simulink model "battery_convertidor_ac_dc_43"  (R2024b)
settings: Solver=FixedStepAuto  StartTime=0.0  StopTime=751  FixedStep=1e-5  RelTol=1e-3
InitFcn:
  | Tint = 1e-5;
  | Ts = 10*Tint;
values from neighbouring files (symbols this model uses):
  C1_filter = 20e-6    (= 2e-05)    [parametros_generales.m]
  I_control = 1    [parametros_generales.m]
  I_control_bat = 5    [parametros_generales.m]
  L_converter = 20e-3    (= 0.02)    [parametros_generales.m]
  Lbat_converter = 1e-5    (= 1e-05)    [parametros_generales.m]
  load_dc = 1000*1000/5    (= 200000)    [parametros_generales.m]
  P_control = 0.01    [parametros_generales.m]
  P_control_bat = 0.7    [parametros_generales.m]
  R = 0.5    [parametros_generales.m]
  R_filter = 0.5    [parametros_generales.m]
  rated_capacitance = 62.5/8    (= 7.8125)    [parametros_generales.m]
  rated_voltage = 144*8    (= 1152)    [parametros_generales.m]
  sample_time_control = 4e-4    (= 0.0004)    [parametros_generales.m]
  voltage_dc_source = 1000    [parametros_generales.m]
undefined symbols (not defined in the file or in its folder): Ion, Lithium
libraries: spsIGBTDiodeLib x24, spsCurrentMeasurementLib x23, spsSeriesRLCBranchLib x20, spsVoltageMeasurementLib x14, spsPower3phInstantaneousLib x8, spsThreePhaseVIMeasurementLib x8, simulink x7, dspstat3 x6, slpidlib x3, spsBatteryLib x2, spsVariableCapacitorLib x1, spsVariableResistorLib x1
(part 2 of 2)

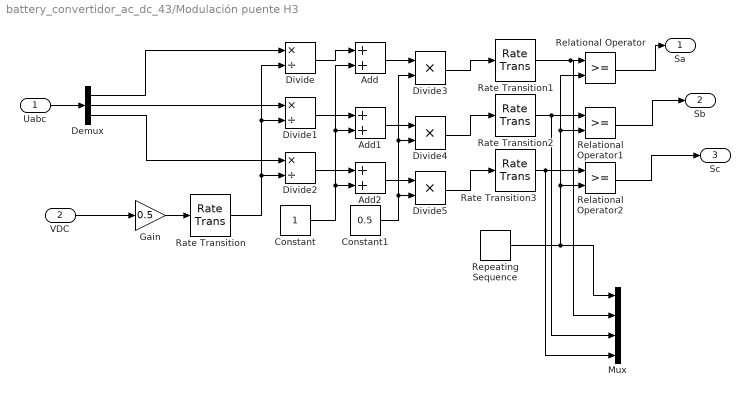
== system battery_convertidor_ac_dc_43/Modulación puente H3 ==
  Uabc : Inport
  VDC : Inport  Port=2
  Add : Sum
  Add1 : Sum
  Add2 : Sum
  Constant : Constant
  Constant1 : Constant  Value=0.5
  Demux : Demux  Outputs=3
  Divide : Product  Inputs=*/
  Divide1 : Product  Inputs=*/
  Divide2 : Product  Inputs=*/
  Divide3 : Product  Inputs=**
  Divide4 : Product  Inputs=**
  Divide5 : Product  Inputs=**
  Gain : Gain  Gain=0.5
  Mux : Mux
  Rate Transition : RateTransition  OutPortSampleTime=Ts
  Rate Transition1 : RateTransition  OutPortSampleTime=Tint
  Rate Transition2 : RateTransition  OutPortSampleTime=Tint
  Rate Transition3 : RateTransition  OutPortSampleTime=Tint
  Relational Operator : RelationalOperator  OutDataTypeStr=boolean  RndMeth=Simplest  InputSameDT=off
  Relational Operator1 : RelationalOperator  OutDataTypeStr=boolean  RndMeth=Simplest  InputSameDT=off
  Relational Operator2 : RelationalOperator  OutDataTypeStr=boolean  RndMeth=Simplest  InputSameDT=off
  Repeating Sequence : simulink/Sources/Repeating Sequence  rep_seq_t=[0 Ts/2 Ts]  rep_seq_y=[0 1 0]
  Sa : Outport
  Sb : Outport  Port=2
  Sc : Outport  Port=3
  wires:
  Demux/3 -> Divide2/1
  Demux/1 -> Divide/1
  Demux/2 -> Divide1/1
  Relational Operator/1 -> Sa/1
  Relational Operator1/1 -> Sb/1
  Relational Operator2/1 -> Sc/1
  Rate Transition/1 -> Divide1/2, Divide/2, Divide2/2
  Divide/1 -> Add/1
  Add/1 -> Divide3/1
  Divide3/1 -> Rate Transition1/1
  Add1/1 -> Divide4/1
  Add2/1 -> Divide5/1
  Divide1/1 -> Add1/1
  Divide4/1 -> Rate Transition2/1
  Divide2/1 -> Add2/1
  Divide5/1 -> Rate Transition3/1
  Constant/1 -> Add2/2, Add1/2, Add/2
  Constant1/1 -> Divide5/2, Divide4/2, Divide3/2
  Uabc/1 -> Demux/1
  Repeating Sequence/1 -> Mux/1, Relational Operator2/2, Relational Operator1/2, Relational Operator/2
  Rate Transition3/1 -> Mux/4, Relational Operator2/1
  Rate Transition2/1 -> Mux/3, Relational Operator1/1
  Rate Transition1/1 -> Mux/2, Relational Operator/1
  Gain/1 -> Rate Transition/1
  VDC/1 -> Gain/1

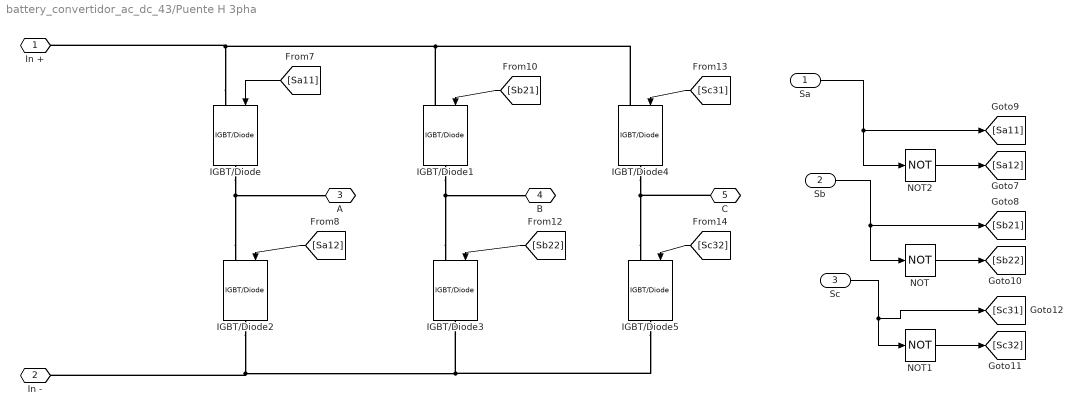
== system battery_convertidor_ac_dc_43/Puente H 3pha ==
  Sa : Inport
  Sb : Inport  Port=2
  Sc : Inport  Port=3
  IGBT/Diode{,1..5} (6 alike) : spsIGBTDiodeLib/IGBT//Diode  Ron=1e-3  Rs=1e5  Cs=inf  Measurements=off
  NOT : Logic  Operator=NOT  IconShape=distinctive  AllPortsSameDT=off  OutDataTypeStr=boolean
  NOT1 : Logic  Operator=NOT  IconShape=distinctive  AllPortsSameDT=off  OutDataTypeStr=boolean
  NOT2 : Logic  Operator=NOT  IconShape=distinctive  AllPortsSameDT=off  OutDataTypeStr=boolean
  In + : PMIOPort  Side=Left
  In - : PMIOPort  Port=2  Side=Left
  A : PMIOPort  Port=3  Side=Right
  B : PMIOPort  Port=4  Side=Right
  C : PMIOPort  Port=5  Side=Right
  wires:
  [Sa11] -> IGBT/Diode/1
  [Sc31] -> IGBT/Diode4/1
  [Sc32] -> IGBT/Diode5/1
  NOT2/1 -> [Sa12]
  NOT/1 -> [Sb22]
  [Sb21] -> IGBT/Diode1/1
  [Sa12] -> IGBT/Diode2/1
  [Sb22] -> IGBT/Diode3/1
  NOT1/1 -> [Sc32]
  Sa/1 -> [Sa11], NOT2/1
  Sb/1 -> [Sb21], NOT/1
  Sc/1 -> [Sc31], NOT1/1
  connections:
  IGBT/Diode2/LConn1 -- A/RConn1 -- IGBT/Diode/RConn1
  IGBT/Diode5/LConn1 -- C/RConn1 -- IGBT/Diode4/RConn1
  In -/RConn1 -- IGBT/Diode2/RConn1 -- IGBT/Diode5/RConn1 -- IGBT/Diode3/RConn1
  IGBT/Diode/LConn1 -- In +/RConn1 -- IGBT/Diode4/LConn1 -- IGBT/Diode1/LConn1
  IGBT/Diode3/LConn1 -- B/RConn1 -- IGBT/Diode1/RConn1

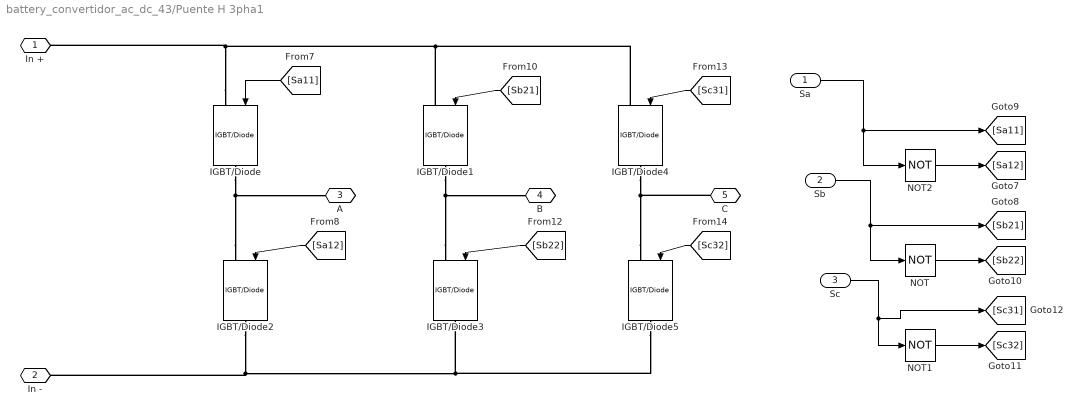
== system battery_convertidor_ac_dc_43/Puente H 3pha1 ==
  Sa : Inport
  Sb : Inport  Port=2
  Sc : Inport  Port=3
  IGBT/Diode{,1..5} (6 alike) : spsIGBTDiodeLib/IGBT//Diode  Ron=1e-3  Rs=1e5  Cs=inf  Measurements=off
  NOT : Logic  Operator=NOT  IconShape=distinctive  AllPortsSameDT=off  OutDataTypeStr=boolean
  NOT1 : Logic  Operator=NOT  IconShape=distinctive  AllPortsSameDT=off  OutDataTypeStr=boolean
  NOT2 : Logic  Operator=NOT  IconShape=distinctive  AllPortsSameDT=off  OutDataTypeStr=boolean
  In + : PMIOPort  Side=Left
  In - : PMIOPort  Port=2  Side=Left
  A : PMIOPort  Port=3  Side=Right
  B : PMIOPort  Port=4  Side=Right
  C : PMIOPort  Port=5  Side=Right
  wires:
  [Sa11] -> IGBT/Diode/1
  [Sc31] -> IGBT/Diode4/1
  [Sc32] -> IGBT/Diode5/1
  NOT2/1 -> [Sa12]
  NOT/1 -> [Sb22]
  [Sb21] -> IGBT/Diode1/1
  [Sa12] -> IGBT/Diode2/1
  [Sb22] -> IGBT/Diode3/1
  NOT1/1 -> [Sc32]
  Sa/1 -> [Sa11], NOT2/1
  Sb/1 -> [Sb21], NOT/1
  Sc/1 -> [Sc31], NOT1/1
  connections:
  IGBT/Diode2/LConn1 -- A/RConn1 -- IGBT/Diode/RConn1
  IGBT/Diode5/LConn1 -- C/RConn1 -- IGBT/Diode4/RConn1
  In -/RConn1 -- IGBT/Diode2/RConn1 -- IGBT/Diode5/RConn1 -- IGBT/Diode3/RConn1
  IGBT/Diode/LConn1 -- In +/RConn1 -- IGBT/Diode4/LConn1 -- IGBT/Diode1/LConn1
  IGBT/Diode3/LConn1 -- B/RConn1 -- IGBT/Diode1/RConn1

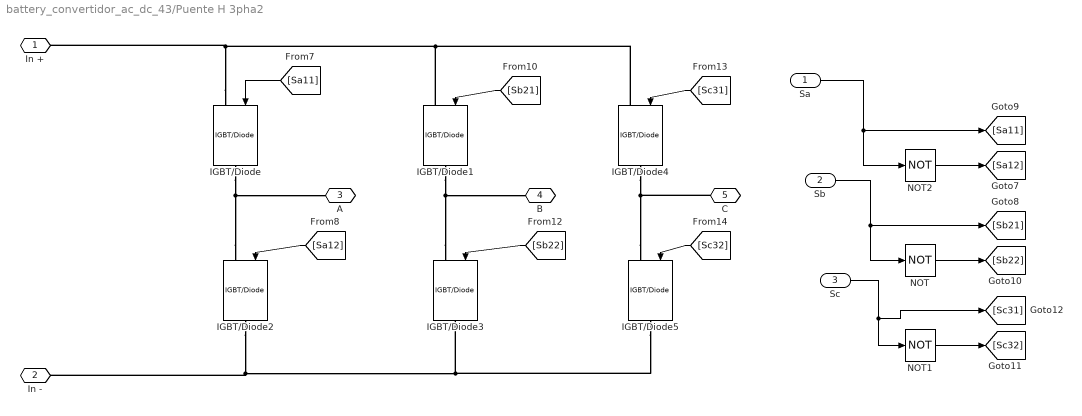
== system battery_convertidor_ac_dc_43/Puente H 3pha2 ==
  Sa : Inport
  Sb : Inport  Port=2
  Sc : Inport  Port=3
  IGBT/Diode{,1..5} (6 alike) : spsIGBTDiodeLib/IGBT//Diode  Ron=1e-3  Rs=1e5  Cs=inf  Measurements=off
  NOT : Logic  Operator=NOT  IconShape=distinctive  AllPortsSameDT=off  OutDataTypeStr=boolean
  NOT1 : Logic  Operator=NOT  IconShape=distinctive  AllPortsSameDT=off  OutDataTypeStr=boolean
  NOT2 : Logic  Operator=NOT  IconShape=distinctive  AllPortsSameDT=off  OutDataTypeStr=boolean
  In + : PMIOPort  Side=Left
  In - : PMIOPort  Port=2  Side=Left
  A : PMIOPort  Port=3  Side=Right
  B : PMIOPort  Port=4  Side=Right
  C : PMIOPort  Port=5  Side=Right
  wires:
  [Sa11] -> IGBT/Diode/1
  [Sc31] -> IGBT/Diode4/1
  [Sc32] -> IGBT/Diode5/1
  NOT2/1 -> [Sa12]
  NOT/1 -> [Sb22]
  [Sb21] -> IGBT/Diode1/1
  [Sa12] -> IGBT/Diode2/1
  [Sb22] -> IGBT/Diode3/1
  NOT1/1 -> [Sc32]
  Sa/1 -> [Sa11], NOT2/1
  Sb/1 -> [Sb21], NOT/1
  Sc/1 -> [Sc31], NOT1/1
  connections:
  IGBT/Diode2/LConn1 -- A/RConn1 -- IGBT/Diode/RConn1
  IGBT/Diode5/LConn1 -- C/RConn1 -- IGBT/Diode4/RConn1
  In -/RConn1 -- IGBT/Diode2/RConn1 -- IGBT/Diode5/RConn1 -- IGBT/Diode3/RConn1
  IGBT/Diode/LConn1 -- In +/RConn1 -- IGBT/Diode4/LConn1 -- IGBT/Diode1/LConn1
  IGBT/Diode3/LConn1 -- B/RConn1 -- IGBT/Diode1/RConn1

== system battery_convertidor_ac_dc_43/Subs switched model  ==
  Pref : Inport
  Vdc : Inport  Port=2
  Current : Inport  Port=3
  L_converter : Inport  Port=4
  CONTROL1 : Subsystem
      settings: PortSchema="{\"entries\":[{\"content\":{\"sides\":[{\"content\":{\"connectorIds\":[\"In1\",\"In2\",\"In3\"]},\"type\":\"ConnectorPlacement.EquallySpacedRectSide\",\"uuid\":\"a9fb8ebe-351f-4a6a-8a99-1a707ba371b7\"},{\"content\":{\"side\":\"RIGHT\"},\"type\":\"ConnectorPlacement.EquallySpacedRectSide\",\"uuid\":\"7ade986f-e35c-4725-83b2-d097e8990248\"},{\"content\":{\"side\":\"TOP\"},\"type\":\"ConnectorPlacement.EquallySpacedRectSide\",\"uuid\":\"4cf2127c-82c5-4c3b-b4b0-71fb60814c91\"},{\"content\":{\"connectorIds\":[\"Out1\"],\"side\":\"BOTTOM\"},\"type\":\"ConnectorPlacement.EquallySpacedRectSide\",\"uuid\":\"8e0559a2-5d7f-4423-aa54-ebeb3f1127a6\"}]},\"type\":\"ConnectorPlacement.EquallySpacedConnector\",\"uuid\":\"11aed1fb-cd52-41ab-8417-ffeb50d501f6\"}],\"packageUris\":[\"http://schema.mathworks.com/mf0/Connector/R2020b\"],\"version\":\"1.0\"}"
  Convertidor : Subsystem
      settings: PortSchema="{\"entries\":[{\"content\":{\"sides\":[{\"content\":{\"connectorIds\":[\"LConn1\",\"LConn2\"]},\"type\":\"ConnectorPlacement.EquallySpacedRectSide\",\"uuid\":\"7a980847-0fd3-4a52-ae22-59cd2a1ed559\"},{\"content\":{\"connectorIds\":[\"RConn1\",\"RConn2\"],\"side\":\"RIGHT\"},\"type\":\"ConnectorPlacement.EquallySpacedRectSide\",\"uuid\":\"85effeeb-73a6-4b0a-b51b-5eb0082317ff\"},{\"content\":{\"connectorIds\":[\"In1\",\"In2\"],\"side\":\"TOP\"},\"type\":\"ConnectorPlacement.EquallySpacedRectSide\",\"uuid\":\"eb55fae0-79ad-414f-ab96-49c332138803\"},{\"content\":{\"side\":\"BOTTOM\"},\"type\":\"ConnectorPlacement.EquallySpacedRectSide\",\"uuid\":\"1fd972ff-419a-4657-8ea4-57d89be2b868\"}]},\"type\":\"ConnectorPlacement.EquallySpacedConnector\",\"uuid\":\"1807473d-fd42-44e0-a7e4-668a7bf21429\"}],\"packageUris\":[\"http://schema.mathworks.com/mf0/Connector/R2020b\"],\"version\":\"1.0\"}"
  + : PMIOPort  Side=Left
  - : PMIOPort  Port=2  Side=Left
  l+ : PMIOPort  Port=3  Side=Right
  l- : PMIOPort  Port=4  Side=Right
  wires:
  Pref/1 -> CONTROL1/1(pref)
  L_converter/1 -> Convertidor/2(L1_converter)
  Current/1 -> CONTROL1/3(current)
  Vdc/1 -> CONTROL1/2(vdc)
  CONTROL1/1(pulse) -> Convertidor/1(S)
  connections:
  +/RConn1 -- Convertidor/LConn1
  Convertidor/RConn2 -- l-/RConn1
  Convertidor/LConn2 -- -/RConn1
  Convertidor/RConn1 -- l+/RConn1

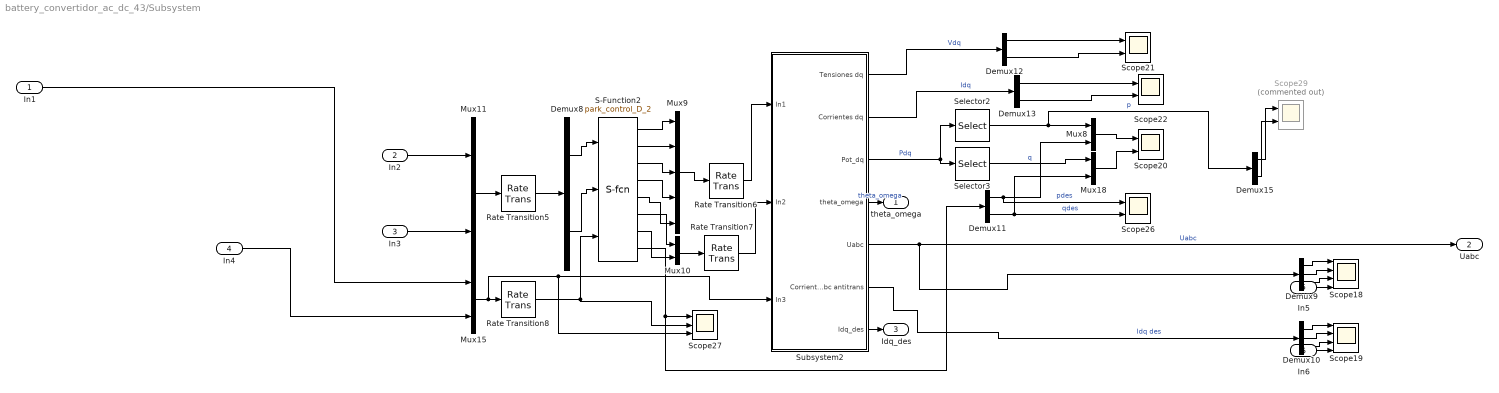
== system battery_convertidor_ac_dc_43/Subsystem ==
  In1 : Inport
  In2 : Inport  Port=2
  In3 : Inport  Port=3
  In4 : Inport  Port=4
  In5 : Inport  Port=5
  In6 : Inport  Port=6
  Demux10 : Demux  Outputs=3
  Demux{8,11..13,15} (5 alike) : Demux  Outputs=2
  Demux9 : Demux  Outputs=3
  Mux{8,10..11,15,18} (5 alike) : Mux  Inputs=2
  Mux9 : Mux  Inputs=5
  Rate Transition5 : RateTransition  OutPortSampleTime=Ts
  Rate Transition6 : RateTransition  Deterministic=off  InitialCondition=[0]  OutPortSampleTime=Tint
  Rate Transition7 : RateTransition  Deterministic=off  InitialCondition=[0]  OutPortSampleTime=Tint
  Rate Transition8 : RateTransition  OutPortSampleTime=Tint
  S-Function2 : S-Function  FunctionName=park_control_D_2  SFunctionDeploymentMode=off  EnableBusSupport=off
  Scope18 : Scope  NumInputPorts=4
  Scope19 : Scope  NumInputPorts=4
  Scope{20..22,26} (4 alike) : Scope  NumInputPorts=2
  Scope27 : Scope  NumInputPorts=3
  Scope29 : Scope  Commented=on  NumInputPorts=2
  Selector2 : Selector  InputPortWidth=4  IndexOptions=Index vector (dialog)  Indices=[1 3]  OutputSizes=1
  Selector3 : Selector  InputPortWidth=4  IndexOptions=Index vector (dialog)  Indices=[2 4]  OutputSizes=1
  Subsystem2 : Subsystem
  theta_omega : Outport
  Uabc : Outport  Port=2
  Idq_des : Outport  Port=3
  wires:
  Subsystem2/3(Pot_dq) -> Selector2/1, Selector3/1  "Pdq"
  Demux13/2 -> Scope22/2
  S-Function2/5 -> Mux9/5
  In6/1 -> Scope19/4
  Selector2/1 -> Demux15/1, Mux8/1  "p"
  In3/1 -> Mux11/2
  S-Function2/8 -> Scope27/1, Demux11/1
  Subsystem2/5(Uabc) -> Uabc/1, Demux9/1  "Uabc"
  S-Function2/6 -> Mux10/1
  Selector3/1 -> Mux18/1  "q"
  Demux15/1 -> Scope29/1
  S-Function2/1 -> Mux9/1
  Demux12/1 -> Scope21/1
  Demux15/2 -> Scope29/2
  Subsystem2/7(Idq_des) -> Idq_des/1
  Demux8/2 -> S-Function2/2
  Demux11/1 -> Scope26/1, Mux8/2  "pdes"
  Demux8/1 -> S-Function2/1
  Rate Transition7/1 -> Subsystem2/2(In2)
  Subsystem2/2(Corrientes dq) -> Demux13/1  "Idq"
  Mux15/1 -> Subsystem2/3(In3), Scope27/3, Rate Transition8/1
  Demux9/2 -> Scope18/2
  Demux10/3 -> Scope19/3
  Mux9/1 -> Rate Transition6/1
  Mux11/1 -> Rate Transition5/1
  Rate Transition8/1 -> S-Function2/3, Scope27/2
  S-Function2/7 -> Mux10/2
  Subsystem2/4(theta_omega) -> theta_omega/1  "theta_omega"
  Demux10/1 -> Scope19/1
  In2/1 -> Mux11/1
  In1/1 -> Mux15/1
  Demux9/3 -> Scope18/3
  S-Function2/3 -> Mux9/3
  S-Function2/4 -> Mux9/4
  Demux13/1 -> Scope22/1
  S-Function2/2 -> Mux9/2
  Mux8/1 -> Scope20/1
  Mux18/1 -> Scope20/2
  Demux10/2 -> Scope19/2
  Subsystem2/1(Tensiones dq) -> Demux12/1  "Vdq"
  Rate Transition5/1 -> Demux8/1
  In4/1 -> Mux15/2
  Mux10/1 -> Rate Transition7/1
  Demux9/1 -> Scope18/1
  Rate Transition6/1 -> Subsystem2/1(In1)
  Subsystem2/6(Corriente abc antitrans) -> Demux10/1  "Idq des"
  Demux12/2 -> Scope21/2
  In5/1 -> Scope18/4
  Demux11/2 -> Scope26/2, Mux18/2  "qdes"

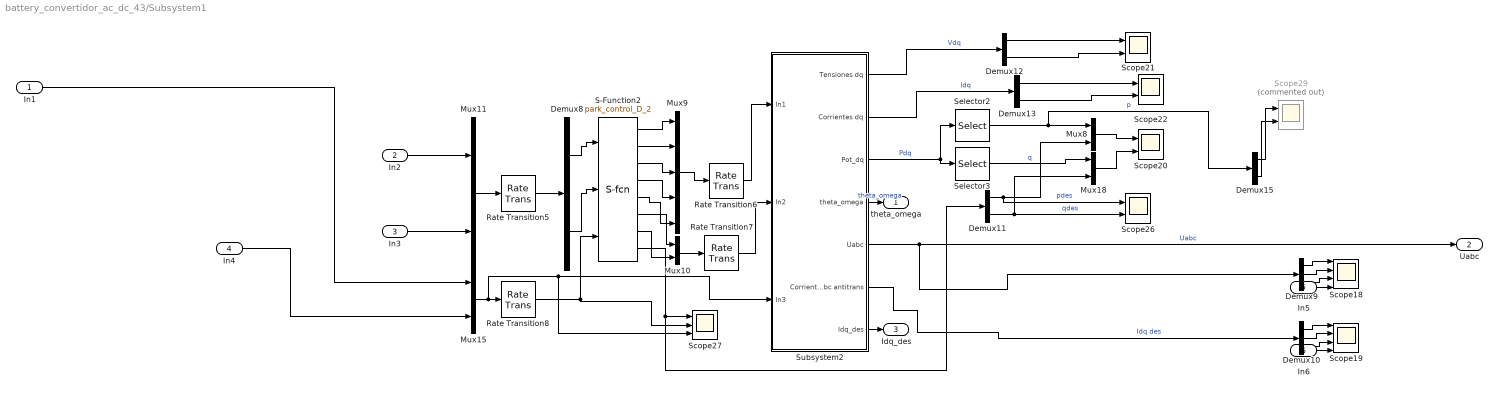
== system battery_convertidor_ac_dc_43/Subsystem1 ==
  In1 : Inport
  In2 : Inport  Port=2
  In3 : Inport  Port=3
  In4 : Inport  Port=4
  In5 : Inport  Port=5
  In6 : Inport  Port=6
  Demux10 : Demux  Outputs=3
  Demux{8,11..13,15} (5 alike) : Demux  Outputs=2
  Demux9 : Demux  Outputs=3
  Mux{8,10..11,15,18} (5 alike) : Mux  Inputs=2
  Mux9 : Mux  Inputs=5
  Rate Transition5 : RateTransition  OutPortSampleTime=Ts
  Rate Transition6 : RateTransition  Deterministic=off  InitialCondition=[0]  OutPortSampleTime=Tint
  Rate Transition7 : RateTransition  Deterministic=off  InitialCondition=[0]  OutPortSampleTime=Tint
  Rate Transition8 : RateTransition  OutPortSampleTime=Tint
  S-Function2 : S-Function  FunctionName=park_control_D_2  SFunctionDeploymentMode=off  EnableBusSupport=off
  Scope18 : Scope  NumInputPorts=4
  Scope19 : Scope  NumInputPorts=4
  Scope{20..22,26} (4 alike) : Scope  NumInputPorts=2
  Scope27 : Scope  NumInputPorts=3
  Scope29 : Scope  Commented=on  NumInputPorts=2
  Selector2 : Selector  InputPortWidth=4  IndexOptions=Index vector (dialog)  Indices=[1 3]  OutputSizes=1
  Selector3 : Selector  InputPortWidth=4  IndexOptions=Index vector (dialog)  Indices=[2 4]  OutputSizes=1
  Subsystem2 : Subsystem
  theta_omega : Outport
  Uabc : Outport  Port=2
  Idq_des : Outport  Port=3
  wires:
  Subsystem2/3(Pot_dq) -> Selector2/1, Selector3/1  "Pdq"
  Demux13/2 -> Scope22/2
  S-Function2/5 -> Mux9/5
  In6/1 -> Scope19/4
  Selector2/1 -> Demux15/1, Mux8/1  "p"
  In3/1 -> Mux11/2
  S-Function2/8 -> Scope27/1, Demux11/1
  Subsystem2/5(Uabc) -> Uabc/1, Demux9/1  "Uabc"
  S-Function2/6 -> Mux10/1
  Selector3/1 -> Mux18/1  "q"
  Demux15/1 -> Scope29/1
  S-Function2/1 -> Mux9/1
  Demux12/1 -> Scope21/1
  Demux15/2 -> Scope29/2
  Subsystem2/7(Idq_des) -> Idq_des/1
  Demux8/2 -> S-Function2/2
  Demux11/1 -> Scope26/1, Mux8/2  "pdes"
  Demux8/1 -> S-Function2/1
  Rate Transition7/1 -> Subsystem2/2(In2)
  Subsystem2/2(Corrientes dq) -> Demux13/1  "Idq"
  Mux15/1 -> Subsystem2/3(In3), Scope27/3, Rate Transition8/1
  Demux9/2 -> Scope18/2
  Demux10/3 -> Scope19/3
  Mux9/1 -> Rate Transition6/1
  Mux11/1 -> Rate Transition5/1
  Rate Transition8/1 -> S-Function2/3, Scope27/2
  S-Function2/7 -> Mux10/2
  Subsystem2/4(theta_omega) -> theta_omega/1  "theta_omega"
  Demux10/1 -> Scope19/1
  In2/1 -> Mux11/1
  In1/1 -> Mux15/1
  Demux9/3 -> Scope18/3
  S-Function2/3 -> Mux9/3
  S-Function2/4 -> Mux9/4
  Demux13/1 -> Scope22/1
  S-Function2/2 -> Mux9/2
  Mux8/1 -> Scope20/1
  Mux18/1 -> Scope20/2
  Demux10/2 -> Scope19/2
  Subsystem2/1(Tensiones dq) -> Demux12/1  "Vdq"
  Rate Transition5/1 -> Demux8/1
  In4/1 -> Mux15/2
  Mux10/1 -> Rate Transition7/1
  Demux9/1 -> Scope18/1
  Rate Transition6/1 -> Subsystem2/1(In1)
  Subsystem2/6(Corriente abc antitrans) -> Demux10/1  "Idq des"
  Demux12/2 -> Scope21/2
  In5/1 -> Scope18/4
  Demux11/2 -> Scope26/2, Mux18/2  "qdes"

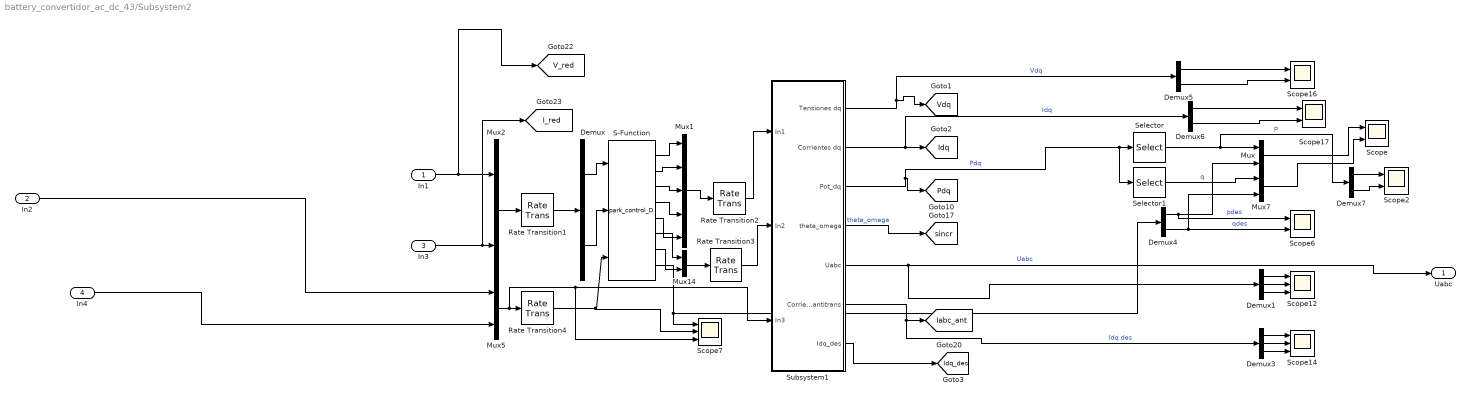
== system battery_convertidor_ac_dc_43/Subsystem2 ==
  In1 : Inport
  In2 : Inport  Port=2
  In3 : Inport  Port=3
  In4 : Inport  Port=4
  Demux{,4..7} (5 alike) : Demux  Outputs=2
  Demux1 : Demux  Outputs=3
  Demux3 : Demux  Outputs=3
  Mux{,2,5,7,14} (5 alike) : Mux  Inputs=2
  Mux1 : Mux  Inputs=5
  Rate Transition1 : RateTransition  OutPortSampleTime=Ts
  Rate Transition2 : RateTransition  Deterministic=off  InitialCondition=[0]  OutPortSampleTime=Tint
  Rate Transition3 : RateTransition  Deterministic=off  InitialCondition=[0]  OutPortSampleTime=Tint
  Rate Transition4 : RateTransition  OutPortSampleTime=Tint
  S-Function : S-Function  FunctionName=park_control_D  SFunctionDeploymentMode=off  EnableBusSupport=off
  Scope{,2,6,16..17} (5 alike) : Scope  NumInputPorts=2
  Scope12 : Scope  NumInputPorts=3
  Scope14 : Scope  NumInputPorts=3
  Scope7 : Scope  NumInputPorts=3
  Selector : Selector  InputPortWidth=4  IndexOptions=Index vector (dialog)  Indices=[1 3]  OutputSizes=1
  Selector1 : Selector  InputPortWidth=4  IndexOptions=Index vector (dialog)  Indices=[2 4]  OutputSizes=1
  Subsystem1 : Subsystem
  Uabc : Outport
  tag scope: I_red=global, Iabc_ant=global, Idq=global, Idq_des=global, Pdq=global, V_red=global, Vdq=global, sincr=global
  wires:
  Subsystem1/5(Uabc) -> Uabc/1, Demux1/1  "Uabc"
  S-Function/8 -> Scope7/1, Demux4/1
  Mux5/1 -> Subsystem1/3(In3), Scope7/3, Rate Transition4/1
  In3/1 -> [I_red], Mux2/2
  S-Function/4 -> Mux1/4
  Demux3/2 -> Scope14/2
  In1/1 -> [V_red], Mux2/1
  Demux7/1 -> Scope2/1
  Demux4/1 -> Scope6/1, Mux/2  "pdes"
  Demux1/3 -> Scope12/3
  Subsystem1/2(Corrientes dq) -> Demux6/1, [Idq]  "Idq"
  Demux6/2 -> Scope17/2
  Demux5/1 -> Scope16/1
  Demux6/1 -> Scope17/1
  Subsystem1/7(Idq_des) -> [Idq_des]
  Demux1/2 -> Scope12/2
  Mux14/1 -> Rate Transition3/1
  Subsystem1/1(Tensiones dq) -> [Vdq], Demux5/1  "Vdq"
  In2/1 -> Mux5/1
  In4/1 -> Mux5/2
  Subsystem1/3(Pot_dq) -> Selector1/1, Selector/1, [Pdq]  "Pdq"
  Demux/1 -> S-Function/1
  Demux3/3 -> Scope14/3
  S-Function/6 -> Mux14/1
  Demux4/2 -> Scope6/2, Mux7/2  "qdes"
  Mux7/1 -> Scope/2
  Subsystem1/4(theta_omega) -> [sincr]  "theta_omega"
  Demux1/1 -> Scope12/1
  Demux7/2 -> Scope2/2
  S-Function/5 -> Mux1/5
  Rate Transition4/1 -> Scope7/2, S-Function/3
  Mux1/1 -> Rate Transition2/1
  Rate Transition2/1 -> Subsystem1/1(In1)
  Mux/1 -> Scope/1
  S-Function/2 -> Mux1/2
  Subsystem1/6(Corriente abc antitrans) -> Demux3/1, [Iabc_ant]  "Idq des"
  Demux/2 -> S-Function/2
  S-Function/1 -> Mux1/1
  Rate Transition3/1 -> Subsystem1/2(In2)
  Demux5/2 -> Scope16/2
  Mux2/1 -> Rate Transition1/1
  S-Function/7 -> Mux14/2
  S-Function/3 -> Mux1/3
  Demux3/1 -> Scope14/1
  Selector/1 -> Demux7/1, Mux/1  "p"
  Rate Transition1/1 -> Demux/1
  Selector1/1 -> Mux7/1  "q"

== system battery_convertidor_ac_dc_43/Subsystem3 ==
  note: 30e-3
  S : Inport
  Current Measurement2 : spsCurrentMeasurementLib/Current Measurement  PhasorSimulation=off  OutputType=Complex  PSBequivalent=0
  IGBT/Diode1 : spsIGBTDiodeLib/IGBT//Diode  Ron=1e-3  Rs=1e5  Cs=inf  Measurements=off
  IGBT/Diode2 : spsIGBTDiodeLib/IGBT//Diode  Ron=1e-3  Rs=1e5  Cs=inf  Measurements=off
  Logical Operator : Logic  Operator=NOT  AllPortsSameDT=off  OutDataTypeStr=boolean
  Series RLC Branch : spsSeriesRLCBranchLib/Series RLC Branch  LConnTagsString=__new0  RConnTagsString=__new0  BranchType=L  Resistance=3  Inductance=Lbat_converter  SetiL0=off  InitialCurrent=0  Capacitance=1e-6  Setx0=off  InitialVoltage=0  Measurements=None
  Series RLC Branch1 : spsSeriesRLCBranchLib/Series RLC Branch  LConnTagsString=__new0  RConnTagsString=__new0  BranchType=L  Resistance=3  Inductance=1e-5  SetiL0=off  InitialCurrent=0  Capacitance=1e-6  Setx0=off  InitialVoltage=0  Measurements=None
  Vin+ : PMIOPort  Side=Left
  Vin- : PMIOPort  Port=2  Side=Left
  Vout+ : PMIOPort  Port=3  Side=Right
  Vout- : PMIOPort  Port=4  Side=Right
  wires:
  Logical Operator/1 -> IGBT/Diode2/1  "S2"
  S/1 -> Logical Operator/1, IGBT/Diode1/1  "S2"
  connections:
  Vout+/RConn1 -- IGBT/Diode2/LConn1
  IGBT/Diode2/RConn1 -- Current Measurement2/RConn1 -- IGBT/Diode1/LConn1
  Vin+/RConn1 -- Series RLC Branch/LConn1
  Series RLC Branch/RConn1 -- Current Measurement2/LConn1
  IGBT/Diode1/RConn1 -- Vout-/RConn1 -- Vin-/RConn1

== system battery_convertidor_ac_dc_43/Subsystem4 ==
  note: 30e-3
  S : Inport
  Current Measurement2 : spsCurrentMeasurementLib/Current Measurement  PhasorSimulation=off  OutputType=Complex  PSBequivalent=0
  IGBT/Diode1 : spsIGBTDiodeLib/IGBT//Diode  Ron=1e-3  Rs=1e5  Cs=inf  Measurements=off
  IGBT/Diode2 : spsIGBTDiodeLib/IGBT//Diode  Ron=1e-3  Rs=1e5  Cs=inf  Measurements=off
  Logical Operator : Logic  Operator=NOT  AllPortsSameDT=off  OutDataTypeStr=boolean
  Series RLC Branch : spsSeriesRLCBranchLib/Series RLC Branch  LConnTagsString=__new0  RConnTagsString=__new0  BranchType=L  Resistance=3  Inductance=Lbat_converter  SetiL0=off  InitialCurrent=0  Capacitance=1e-6  Setx0=off  InitialVoltage=0  Measurements=None
  Series RLC Branch1 : spsSeriesRLCBranchLib/Series RLC Branch  LConnTagsString=__new0  RConnTagsString=__new0  BranchType=L  Resistance=3  Inductance=1e-5  SetiL0=off  InitialCurrent=0  Capacitance=1e-6  Setx0=off  InitialVoltage=0  Measurements=None
  Vin+ : PMIOPort  Side=Left
  Vin- : PMIOPort  Port=2  Side=Left
  Vout+ : PMIOPort  Port=3  Side=Right
  Vout- : PMIOPort  Port=4  Side=Right
  wires:
  Logical Operator/1 -> IGBT/Diode2/1  "S2"
  S/1 -> Logical Operator/1, IGBT/Diode1/1  "S2"
  connections:
  Vout+/RConn1 -- IGBT/Diode2/LConn1
  IGBT/Diode2/RConn1 -- Current Measurement2/RConn1 -- IGBT/Diode1/LConn1
  Vin+/RConn1 -- Series RLC Branch/LConn1
  Series RLC Branch/RConn1 -- Current Measurement2/LConn1
  IGBT/Diode1/RConn1 -- Vout-/RConn1 -- Vin-/RConn1

== system battery_convertidor_ac_dc_43/Subs switched model /CONTROL1 ==
  pref : Inport
  vdc : Inport  Port=2
  current : Inport  Port=3
  Divide2 : Product  Inputs=*/  RndMeth=Zero  SaturateOnIntegerOverflow=on
  PIDC1 : slpidlib/PID Controller  Controller=PI  Form=Parallel  TimeDomain=Discrete-time  UseExternalTs=off  SampleTime=sample_time_control  IntegratorMethod=Forward Euler  FilterMethod=Forward Euler  ControllerParametersSource=internal  P=P_control  I=I_control  UseKiTs=off  D=0  UseExternalDerivativeSource=off  N=100  UseFilter=on  TunerSelectOption=Transfer Function Based (PID Tuner App)  InitialConditionSource=internal  InitialConditionForIntegrator=0.76  InitialConditionForFilter=0  DifferentiatorICPrevScaledInput=0  ExternalReset=none  TrackingMode=off  Kt=1  LimitOutput=on  SatLimitsSource=internal  UpperSaturationLimit=0.99  LowerSaturationLimit=0  LinearizeAsGain=on  AntiWindupMode=clamping  Kb=1  LimitIntegrator=off  UpperIntegratorSaturationLimit=inf  LowerIntegratorSaturationLimit=-inf  POutMin=[]  POutMax=[]  IOutMin=[]  IOutMax=[]  DOutMin=[]  DOutMax=[]  NOutMin=[]  NOutMax=[]  SumOutMin=[]  SumOutMax=[]  SaturationOutMin=[]  SaturationOutMax=[]  PParamMin=[]  PParamMax=[]  IParamMin=[]  IParamMax=[]  DParamMin=[]  DParamMax=[]  NParamMin=[]  NParamMax=[]  KbParamMin=[]  KbParamMax=[]  KtParamMin=[]  KtParamMax=[]  KbOutMin=[]  KbOutMax=[]  KtOutMin=[]  KtOutMax=[]  IntegratorOutMin=[]  IntegratorOutMax=[]  FilterOutMin=[]  FilterOutMax=[]  SumI1OutMin=[]  SumI1OutMax=[]  SumI2OutMin=[]  SumI2OutMax=[]  SumI3OutMin=[]  SumI3OutMax=[]  SumI4OutMin=[]  SumI4OutMax=[]  SumDOutMin=[]  SumDOutMax=[]  DifferentiatorOutMin=[]  DifferentiatorOutMax=[]  FilterDiffOutCoefMin=[]  FilterDiffOutCoefMax=[]  ReciprocalOutMin=[]  ReciprocalOutMax=[]  SumDenOutMin=[]  SumDenOutMax=[]  SumNumOutMin=[]  SumNumOutMax=[]  DivideOutMin=[]  DivideOutMax=[]  UdiffTsProdOutMin=[]  UdiffTsProdOutMax=[]  NTsProdOutMin=[]  NTsProdOutMax=[]  UintegralTsProdOutMin=[]  UintegralTsProdOutMax=[]  UngainTsProdOutMin=[]  UngainTsProdOutMax=[]  ClampingZeroOutDataTypeStr=Inherit: Inherit via back propagation  ClampingZeroOutMin=[]  ClampingZeroOutMax=[]  FilterDenConstantOutDataTypeStr=Inherit: Inherit via back propagation  FilterDenConstantOutMin=[]  FilterDenConstantOutMax=[]  PCopyOutDataTypeStr=Inherit: Inherit via back propagation  PCopyOutMin=[]  PCopyOutMax=[]  NCopyOutDataTypeStr=Inherit: Inherit via back propagation  NCopyOutMin=[]  NCopyOutMax=[]  IntegratorContinuousStateAttributes=''  IntegratorStateMustResolveToSignalObject=off  IntegratorRTWStateStorageClass=Auto  FilterContinuousStateAttributes=''  FilterStateMustResolveToSignalObject=off  FilterRTWStateStorageClass=Auto  ParallelPVariant=InternalParameters  IdealPVariant=Disabled  IVariant=InternalParameters  DVariant=Disabled  IntegratorVariant=Discrete  SatVariant=Enabled  AWVariant=DiscClampingParallel  PCopyVariant=Disabled  TRVariant=Disabled  FdbkBlocksVariant=Forward  IdealPFdbkVariant=Disabled  SatFdbkVariant=Disabled  DerivativeFilterVariant=Disabled  NVariant=Disabled  NCopyVariant=Disabled_SignalSpec  FilterICVariant=Disabled  IntegratorICVariant=InternalICs  ExternalResetVariant=Disabled  TRSumVariant=Passthrough  SumFdbkVariant=Disabled  SumVariant=Sum_PI  TsampFilterVariant=InternalTs  TsampNgainVariant=Passthrough  TsampIntegralVariant=Disabled_SignalSpec  ExternalSaturationOutDataTypeStr=Inherit: Same as second input  DerivativeSourceVariant=Disabled  PreIntVariant=InternalPreInt
  Relational Operator4 : RelationalOperator  OutDataTypeStr=boolean  InputSameDT=off
  Repeating Sequence3 : simulink/Sources/Repeating Sequence  rep_seq_t=[0 Ts/2 Ts]  rep_seq_y=[0 1 0]
  Scope2 : Scope  NumInputPorts=4
  Scope3 : Scope  NumInputPorts=4
  Sum6 : Sum  Inputs=|+-
  pulse : Outport
  wires:
  Sum6/1 -> PIDC1/1, Scope3/3  "I_B_Actuation"
  Repeating Sequence3/1 -> Relational Operator4/2, Scope2/2
  Divide2/1 -> Sum6/1, Scope3/2
  PIDC1/1 -> Scope3/4, Relational Operator4/1  "I_B_Actuation"
  Relational Operator4/1 -> pulse/1, Scope2/3  "pulse"
  vdc/1 -> Divide2/2
  current/1 -> Sum6/2
  pref/1 -> Divide2/1

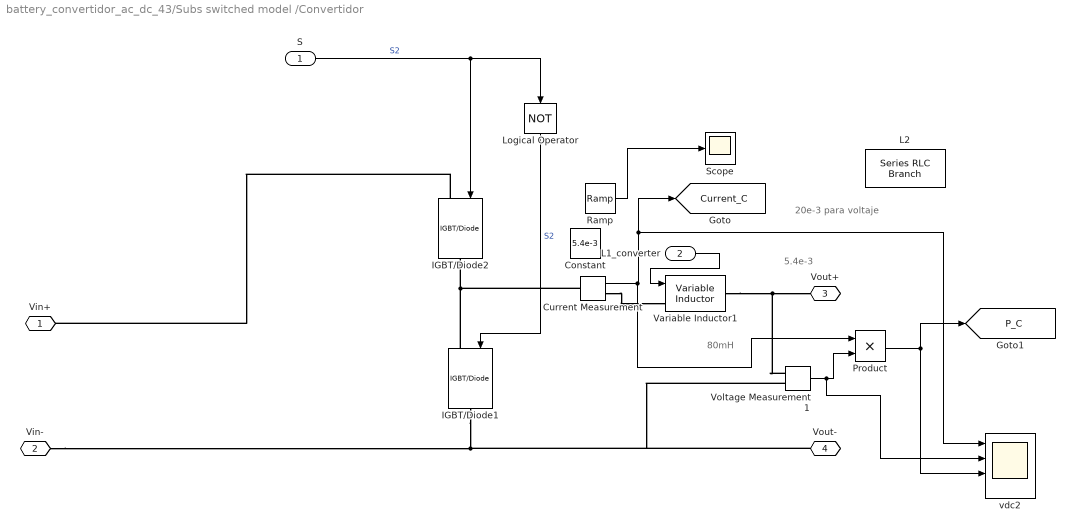
== system battery_convertidor_ac_dc_43/Subs switched model /Convertidor ==
  note: 20e-3 para voltaje
  note: 5.4e-3
  note: 80mH
  S : Inport
  L1_converter : Inport  Port=2
  Constant : Constant  Value=5.4e-3
  Current Measurement : spsCurrentMeasurementLib/Current Measurement  PhasorSimulation=off  OutputType=Complex  PSBequivalent=0
  IGBT/Diode1 : spsIGBTDiodeLib/IGBT//Diode  Ron=1e-3  Rs=1e5  Cs=inf  Measurements=off
  IGBT/Diode2 : spsIGBTDiodeLib/IGBT//Diode  Ron=1e-3  Rs=1e5  Cs=inf  Measurements=off
  L2 : spsSeriesRLCBranchLib/Series RLC Branch  LConnTagsString=__new0  RConnTagsString=__new0  BranchType=L  Resistance=3  Inductance=2.4e-3  SetiL0=off  InitialCurrent=0  Capacitance=1e-6  Setx0=off  InitialVoltage=0  Measurements=None
  Logical Operator : Logic  Operator=NOT  AllPortsSameDT=off  OutDataTypeStr=boolean
  Product : Product
  Ramp : simulink/Sources/Ramp  slope=15e-3  start=0  InitialOutput=3.5e-3
  Scope : Scope
  Variable Inductor1 : spsVariableInductorLib/Variable Inductor  methode=Backward Euler  Labsmin=1e-6  Initialize=off  iL0=0  L0=1e-3  Vl0=-424.0003
  Voltage Measurement1 : spsVoltageMeasurementLib/Voltage Measurement  PhasorSimulation=off  OutputType=Complex  PSBequivalent=0
  vdc2 : Scope  NumInputPorts=4
  Vin+ : PMIOPort  Side=Left
  Vin- : PMIOPort  Port=2  Side=Left
  Vout+ : PMIOPort  Port=3  Side=Right
  Vout- : PMIOPort  Port=4  Side=Right
  tag scope: Current_C=global, P_C=global
  wires:
  S/1 -> IGBT/Diode2/1, Logical Operator/1  "S2"
  Logical Operator/1 -> IGBT/Diode1/1  "S2"
  Current Measurement/1 -> Product/1, vdc2/1, [Current_C]
  Voltage Measurement1/1 -> vdc2/2, Product/2
  Product/1 -> [P_C], vdc2/3
  Ramp/1 -> Scope/1
  L1_converter/1 -> Variable Inductor1/1
  connections:
  Vin-/RConn1 -- Voltage Measurement1/LConn2 -- Vout-/RConn1 -- IGBT/Diode1/RConn1
  IGBT/Diode1/LConn1 -- Current Measurement/LConn1 -- IGBT/Diode2/RConn1
  IGBT/Diode2/LConn1 -- Vin+/RConn1
  Voltage Measurement1/LConn1 -- Variable Inductor1/RConn1 -- Vout+/RConn1
  Current Measurement/RConn1 -- Variable Inductor1/LConn1

== system battery_convertidor_ac_dc_43/Subsystem/Subsystem2 ==
  In1 : Inport
  In2 : Inport  Port=2
  In3 : Inport  Port=3
  Constant : Constant  Value=7
  Constant1 : Constant  Value=-7
  Demux1 : Demux  Outputs=5
  Demux2 : Demux  Outputs=2
  Mux : Mux  Inputs=3
  Mux1 : Mux  Inputs=2
  Mux2 : Mux  Inputs=2
  Tensiones dq : Outport
  Corrientes dq : Outport  Port=2
  Pot_dq : Outport  Port=3
  theta_omega : Outport  Port=4
  Uabc : Outport  Port=5
  Corriente abc antitrans : Outport  Port=6
  Idq_des : Outport  Port=7
  wires:
  Mux/1 -> Tensiones dq/1  "Tensiones dq"
  Constant1/1 -> Mux/3
  Constant/1 -> Mux/2
  Demux1/1 -> Mux/1
  In1/1 -> Demux1/1
  Demux2/1 -> Uabc/1
  Demux2/2 -> Corriente abc antitrans/1
  In2/1 -> Demux2/1
  Demux1/4 -> theta_omega/1
  Demux1/5 -> Mux2/2, Idq_des/1
  Mux1/1 -> Pot_dq/1  "Pot_dq dq"
  Demux1/3 -> Mux1/1  "Pots_alf_bet"
  In3/1 -> Mux1/2
  Mux2/1 -> Corrientes dq/1  "Pot_dq dq"
  Demux1/2 -> Mux2/1  "Corrientes dq"

== system battery_convertidor_ac_dc_43/Subsystem1/Subsystem2 ==
  In1 : Inport
  In2 : Inport  Port=2
  In3 : Inport  Port=3
  Constant : Constant  Value=7
  Constant1 : Constant  Value=-7
  Demux1 : Demux  Outputs=5
  Demux2 : Demux  Outputs=2
  Mux : Mux  Inputs=3
  Mux1 : Mux  Inputs=2
  Mux2 : Mux  Inputs=2
  Tensiones dq : Outport
  Corrientes dq : Outport  Port=2
  Pot_dq : Outport  Port=3
  theta_omega : Outport  Port=4
  Uabc : Outport  Port=5
  Corriente abc antitrans : Outport  Port=6
  Idq_des : Outport  Port=7
  wires:
  Mux/1 -> Tensiones dq/1  "Tensiones dq"
  Constant1/1 -> Mux/3
  Constant/1 -> Mux/2
  Demux1/1 -> Mux/1
  In1/1 -> Demux1/1
  Demux2/1 -> Uabc/1
  Demux2/2 -> Corriente abc antitrans/1
  In2/1 -> Demux2/1
  Demux1/4 -> theta_omega/1
  Demux1/5 -> Mux2/2, Idq_des/1
  Mux1/1 -> Pot_dq/1  "Pot_dq dq"
  Demux1/3 -> Mux1/1  "Pots_alf_bet"
  In3/1 -> Mux1/2
  Mux2/1 -> Corrientes dq/1  "Pot_dq dq"
  Demux1/2 -> Mux2/1  "Corrientes dq"

== system battery_convertidor_ac_dc_43/Subsystem2/Subsystem1 ==
  In1 : Inport
  In2 : Inport  Port=2
  In3 : Inport  Port=3
  Constant : Constant  Value=7
  Constant1 : Constant  Value=-7
  Demux1 : Demux  Outputs=5
  Demux2 : Demux  Outputs=2
  Mux : Mux  Inputs=3
  Mux1 : Mux  Inputs=2
  Mux2 : Mux  Inputs=2
  Tensiones dq : Outport
  Corrientes dq : Outport  Port=2
  Pot_dq : Outport  Port=3
  theta_omega : Outport  Port=4
  Uabc : Outport  Port=5
  Corriente abc antitrans : Outport  Port=6
  Idq_des : Outport  Port=7
  wires:
  Mux/1 -> Tensiones dq/1  "Tensiones dq"
  Constant1/1 -> Mux/3
  Constant/1 -> Mux/2
  Demux1/1 -> Mux/1
  In1/1 -> Demux1/1
  Demux2/1 -> Uabc/1
  Demux2/2 -> Corriente abc antitrans/1
  In2/1 -> Demux2/1
  Demux1/4 -> theta_omega/1
  Demux1/5 -> Mux2/2, Idq_des/1
  Mux1/1 -> Pot_dq/1  "Pot_dq dq"
  Demux1/3 -> Mux1/1  "Pots_alf_bet"
  In3/1 -> Mux1/2
  Mux2/1 -> Corrientes dq/1  "Pot_dq dq"
  Demux1/2 -> Mux2/1  "Corrientes dq"

== matlab function battery_convertidor_ac_dc_43/MATLAB Function1 ==
  data: P_carga_ac input; P_bateria output; P_carga_dc input; Per_batt input; P_ultracapacitor output; P_smes output; P_ac_dc output; Per_ultra input; Per_smes input; Per_ac_dc input
function [P_bateria, P_ultracapacitor, P_smes, P_ac_dc] = gestion_energia(P_carga_ac, P_carga_dc,Per_batt,Per_ultra,Per_smes,Per_ac_dc)
    % P_carga_ac: Potencia de carga en AC (en W)
    % P_carga_dc: Potencia de carga en DC (en W)
    
    % Parámetros de los sistemas
    % Inicializar las salidas
    P_bateria = 0;
    P_ultracapacitor = 0;
    P_smes = 0;
    P_ac_dc = 0;
    
    % Gestionar la potencia AC de la carga
    if P_carga_ac >= 0
        % Intentar abastecer la carga con la batería e inversor
        P_bateria = Per_batt;  % Potencia máxima que la batería puede proporcionar 
        if P_bateria >= P_carga_ac
            P_faltante_ac=0;
            P_sobrante_ac=P_bateria-P_carga_ac;
        else
            P_faltante_ac = P_carga_ac - P_bateria; % El resto lo cubre la red externa
            P_sobrante_ac=0;
        end
    end
    
    % Gestionar la potencia DC de la carga
    if P_carga_dc >= 0
        potencia_dc_total=Per_ultra+Per_smes+Per_ac_dc;
          P_ultracapacitor =Per_ultra;
          P_smes = Per_smes;
          P_ac_dc =Per_ac_dc;
        if potencia_dc_total>= P_carga_dc
            P_sobrante_dc=potencia_dc_total-P_carga_dc;
            P_faltante_dc=0;
        else
            P_faltante_dc=P_carga_dc-potencia_dc_total;
            P_sobrante_dc=0;
        end
    end

== matlab function battery_convertidor_ac_dc_43/MATLAB Function ==
  data: P_carga_ac input; P_bateria output; P_carga_dc input; Per_batt input; P_ultracapacitor output; P_smes output; P_red_externa output; Per_ultra input; Per_smes input; Per_red input
function [P_bateria, P_ultracapacitor, P_smes, P_red_externa] = gestion_energia(P_carga_ac, P_carga_dc,Per_batt,Per_ultra,Per_smes,Per_red)
    % P_carga_ac: Potencia de carga en AC (en W)
    % P_carga_dc: Potencia de carga en DC (en W)
    
    % Parámetros de los sistemas
    % Inicializar las salidas
    P_bateria = 0;
    P_ultracapacitor = 0;
    P_smes = 0;
    P_faltante = 0;
    P_red_externa = 0;
    
    % Gestionar la potencia AC de la carga
    if P_carga_ac > 0
        % Intentar abastecer la carga con la batería e inversor
        potencia_bateria = (Per_batt / 100) * P_carga_ac; % Potencia máxima que la batería puede proporcionar 
        if potencia_bateria >= P_carga_ac
            P_bateria = (Per_batt/100)*P_carga_ac; % La batería cubre toda la carga AC
            P_faltante=0;
        else
            P_bateria = potencia_bateria; % La batería cubre solo la potencia que puede
            P_faltante = P_carga_ac - P_bateria; % El resto lo cubre la red externa
        end
    end
    
    % Gestionar la potencia DC de la carga
    if P_carga_dc > 0
          P_ultracapacitor =(Per_ultra/100)*P_carga_dc;
          P_smes = (Per_smes/100)*P_carga_dc;
          P_red_externa =(Per_red/100)*P_carga_dc+P_faltante;%% aqui le sumo la potencia faltante a la red externa , pero se puede sumar al smes o ultrcap
    end
